simulink model "Protection"  (R2023b)
settings: Solver=FixedStepAuto  StartTime=0.0  StopTime=2  RelTol=1e-3
InitFcn:
  | Ts_Control=100e-6;
  | fs=50000;
  | Ts=1/fs/10;
  | Ts_Power=Ts;
  | Ts_control=5*Ts;
  | wnom=314.16;
  | Lf=5e-3;
  | Rf=0.1;
  | Cf=50e-6;
  | 
  | 
  | % choosing crossover frequency
  | fc=(1/10)*fs;
  | wc=2*pi*fc;
  | Ti=1/wc;
  | Kpc=Lf/Ti;
  | 
  | Kic=Rf/Ti;
  | 
  | x=[837.555 8.2389 0.057896 268.1361 0.74685 242.918 0.062838 291.0935]
  | 
  | 
  | Kvi=x(1);Kvp=x(2);Kcp=x(3);Kci=x(4);
  | Kvpb=x(5);Kvib=x(6);Kcpb=x(7);Kcib=x(8);
  | 
  | 
  | x1=[0.202905850069502  0.158544693742674   0.10408       75.97091  837.555350377473 8.2389271001531  0.10408       75.97091];
  | 
  | Kvif=x1(1);Kvpf=x1(2);Kcpf=x1(3);Kcif=x1(4);
  | Kvim=x1(5);Kvpm=x1(6);Kcpm=x1(7);Kcim=x1(8);
undefined symbols (not defined in the file): D1, Delta, Hydride, Metal, Nickel, sigbuilder_block
libraries: spsSeriesRLCBranchLib x52, spsVoltageMeasurementLib x22, powerlib_extras x18, spsCurrentMeasurementLib x13, spsIdealSwitchLib x12, simulink x8, slpidlib x7, spsGroundLib x6, spsBreakerLib x5, spsDiodeLib x4, spsIGBTLib x4, spsThreePhaseVIMeasurementLib x4
(part 2 of 2)

== system Protection/PV 1/MPPT ==
  In1 : Inport
  In2 : Inport  Port=2
  Add1 : Sum  Inputs=-+
  Constant1 : Constant  Value=0
  Constant2 : Constant  Value=0.5
  Constant3 : Constant
  MPPT : Subsystem
  Relational Operator : RelationalOperator  Operator=<  OutDataTypeStr=boolean  InputSameDT=off
  Repeating Sequence : simulink/Sources/Repeating Sequence  rep_seq_t=[0 0.00005 0.0001]  rep_seq_y=[0 1 0]
  Sign : Signum
  Switch2 : Switch  Criteria=u2 > Threshold  SaturateOnIntegerOverflow=off  InputSameDT=off
  Unit Delay1 : UnitDelay  SampleTime=2e-6  HasFrameUpgradeWarning=on
  Unit Delay2 : UnitDelay  SampleTime=2e-6  HasFrameUpgradeWarning=on
  Out1 : Outport
  wires:
  Relational Operator/1 -> Out1/1
  Repeating Sequence/1 -> Relational Operator/2
  Add1/1 -> Relational Operator/1
  Constant2/1 -> Add1/2
  In2/1 -> Unit Delay2/1
  In1/1 -> Unit Delay1/1
  Switch2/1 -> Add1/1
  Constant3/1 -> Switch2/3
  Sign/1 -> Switch2/2
  Constant1/1 -> Switch2/1
  Unit Delay2/1 -> MPPT/2(I_PV)
  Unit Delay1/1 -> MPPT/1(V_PV)
  MPPT/1(sign) -> Sign/1

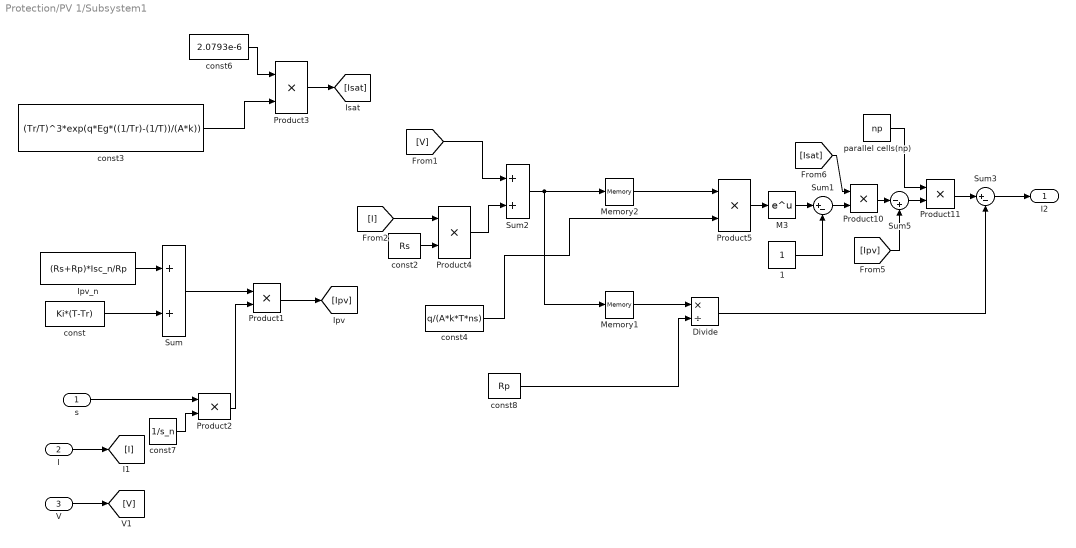
== system Protection/PV 1/Subsystem1 ==
  s : Inport
  I : Inport  Port=2
  V : Inport  Port=3
  1 : Constant
  Divide : Product  Inputs=*/
  Ipv_n : Constant  Value=(Rs+Rp)*Isc_n/Rp
  M3 : Math  SignedPower=on
  Memory1 : Memory
  Memory2 : Memory
  Product{1..5,10..11} (7 alike) : Product  RndMeth=Zero
  Sum : Sum
  Sum1 : Sum  Inputs=|+-
  Sum2 : Sum
  Sum3 : Sum  Inputs=|+-
  Sum5 : Sum  Inputs=|-+
  const : Constant  Value=Ki*(T-Tr)
  const2 : Constant  Value=Rs
  const3 : Constant  Value=(Tr/T)^3*exp(q*Eg*((1/Tr)-(1/T))/(A*k))
  const4 : Constant  Value=q/(A*k*T*ns)
  const6 : Constant  Value=2.0793e-6
  const7 : Constant  Value=1/s_n
  const8 : Constant  Value=Rp
  parallel cells(np) : Constant  Value=np
  I2 : Outport
  wires:
  Memory2/1 -> Product5/1
  Memory1/1 -> Divide/1
  Divide/1 -> Sum3/2
  Sum3/1 -> I2/1
  Product11/1 -> Sum3/1
  const8/1 -> Divide/2
  Ipv_n/1 -> Sum/1
  Product4/1 -> Sum2/2
  const7/1 -> Product2/2
  s/1 -> Product2/1
  Product2/1 -> Product1/2
  Sum2/1 -> Memory1/1, Memory2/1
  parallel cells(np)/1 -> Product11/1
  Sum5/1 -> Product11/2
  Product10/1 -> Sum5/1
  [Ipv] -> Sum5/2
  [Isat] -> Product10/1
  Sum1/1 -> Product10/2
  1/1 -> Sum1/2
  M3/1 -> Sum1/1
  Product5/1 -> M3/1
  const4/1 -> Product5/2
  [I] -> Product4/1
  const2/1 -> Product4/2
  [V] -> Sum2/1
  I/1 -> [I]
  V/1 -> [V]
  Product3/1 -> [Isat]
  const3/1 -> Product3/2
  Product1/1 -> [Ipv]
  Sum/1 -> Product1/1
  const/1 -> Sum/2
  const6/1 -> Product3/1

== system Protection/Subsystem/CPL1 ==
  2 : powerlib_extras/Control  Blocks/1st-Order  Filter  FilterType=Lowpass  Tc=2e-3  Initialize=off  Vac_Init=[0.8 -25 60]  Vdc_Init=-0.4  PlotResponse=off  param1=[1 500 1]
  Current Measurement : spsCurrentMeasurementLib/Current Measurement  PhasorSimulation=off  OutputType=Complex  PSBequivalent=0
  Diode1 : spsDiodeLib/Diode  Ron=0.001  Lon=0  Vf=0.8  IC=0  UseSnubber=off  Rs=500  Cs=250e-9  Measurements=off
  Display2 : Display
  Display3 : Display
  Display4 : Display
  IGBT : spsIGBTLib/IGBT  Ron=0.001  Lon=0  Vf=1  Tf=1e-6  Tt=2e-6  IC=0  Rs=1e5  Cs=inf  Measurements=on
  Product1 : Product  RndMeth=Zero
  SLB : spsSeriesRLCBranchLib/Series RLC Branch  LConnTagsString=__new0  RConnTagsString=__new0  BranchType=RL  Resistance=0.01  Inductance=9.2e-3  SetiL0=off  InitialCurrent=0  Capacitance=1e-6  Setx0=off  InitialVoltage=0  Measurements=Branch current
  Scope2 : Scope  NumInputPorts=2
  Subsystem : Subsystem
  Terminator : Terminator
  Unit Delay : UnitDelay  SampleTime=-1  HasFrameUpgradeWarning=on
  Voltage Measurement : spsVoltageMeasurementLib/Voltage Measurement  PhasorSimulation=off  OutputType=Complex  PSBequivalent=0
  Voltage Measurement1 : spsVoltageMeasurementLib/Voltage Measurement  PhasorSimulation=off  OutputType=Complex  PSBequivalent=0
  dc link1 : spsSeriesRLCBranchLib/Series RLC Branch  LConnTagsString=__new0  RConnTagsString=__new0  BranchType=C  Resistance=1  Inductance=1e-3  SetiL0=off  InitialCurrent=0  Capacitance=5000e-6  Setx0=on  InitialVoltage=240  Measurements=None
  Vout+ : PMIOPort  Tag=PMCPort  Side=Right
  Vout_ : PMIOPort  Tag=PMCPort  Port=2  Side=Right
  +Vin : PMIOPort  Tag=PMCPort  Port=3  Side=Left
  _Vin : PMIOPort  Tag=PMCPort  Port=4  Side=Left
  wires:
  Voltage Measurement1/1 -> Display4/1
  IGBT/1 -> Terminator/1
  Current Measurement/1 -> Subsystem/1(IL), Display3/1, Product1/2
  Voltage Measurement/1 -> Product1/1, Scope2/1, Subsystem/2(Vdc), Display2/1
  Subsystem/1(Out2) -> Unit Delay/1
  Unit Delay/1 -> IGBT/1
  Product1/1 -> 2/1
  2/1 -> Scope2/2
  connections:
  Diode1/LConn1 -- _Vin/RConn1 -- Voltage Measurement1/LConn2 -- Voltage Measurement/LConn2 -- Vout_/RConn1 -- dc link1/RConn1
  Current Measurement/LConn1 -- SLB/RConn1
  IGBT/RConn1 -- Diode1/RConn1 -- SLB/LConn1
  dc link1/LConn1 -- Current Measurement/RConn1 -- Voltage Measurement/LConn1 -- Vout+/RConn1
  Voltage Measurement1/LConn1 -- IGBT/LConn1 -- +Vin/RConn1

== system Protection/Subsystem1/CPL1 ==
  2 : powerlib_extras/Control  Blocks/1st-Order  Filter  FilterType=Lowpass  Tc=2e-3  Initialize=off  Vac_Init=[0.8 -25 60]  Vdc_Init=-0.4  PlotResponse=off  param1=[1 500 1]
  Current Measurement : spsCurrentMeasurementLib/Current Measurement  PhasorSimulation=off  OutputType=Complex  PSBequivalent=0
  Diode1 : spsDiodeLib/Diode  Ron=0.001  Lon=0  Vf=0.8  IC=0  UseSnubber=off  Rs=500  Cs=250e-9  Measurements=off
  Display2 : Display
  Display3 : Display
  Display4 : Display
  IGBT : spsIGBTLib/IGBT  Ron=0.001  Lon=0  Vf=1  Tf=1e-6  Tt=2e-6  IC=0  Rs=1e5  Cs=inf  Measurements=on
  Product1 : Product  RndMeth=Zero
  SLB : spsSeriesRLCBranchLib/Series RLC Branch  LConnTagsString=__new0  RConnTagsString=__new0  BranchType=RL  Resistance=0.01  Inductance=9.2e-3  SetiL0=off  InitialCurrent=0  Capacitance=1e-6  Setx0=off  InitialVoltage=0  Measurements=Branch current
  Scope2 : Scope  NumInputPorts=2
  Subsystem : Subsystem
  Terminator : Terminator
  Unit Delay : UnitDelay  SampleTime=-1  HasFrameUpgradeWarning=on
  Voltage Measurement : spsVoltageMeasurementLib/Voltage Measurement  PhasorSimulation=off  OutputType=Complex  PSBequivalent=0
  Voltage Measurement1 : spsVoltageMeasurementLib/Voltage Measurement  PhasorSimulation=off  OutputType=Complex  PSBequivalent=0
  dc link1 : spsSeriesRLCBranchLib/Series RLC Branch  LConnTagsString=__new0  RConnTagsString=__new0  BranchType=C  Resistance=1  Inductance=1e-3  SetiL0=off  InitialCurrent=0  Capacitance=5000e-6  Setx0=on  InitialVoltage=240  Measurements=None
  Vout+ : PMIOPort  Tag=PMCPort  Side=Right
  Vout_ : PMIOPort  Tag=PMCPort  Port=2  Side=Right
  +Vin : PMIOPort  Tag=PMCPort  Port=3  Side=Left
  _Vin : PMIOPort  Tag=PMCPort  Port=4  Side=Left
  wires:
  Voltage Measurement1/1 -> Display4/1
  IGBT/1 -> Terminator/1
  Current Measurement/1 -> Subsystem/1(IL), Display3/1, Product1/2
  Voltage Measurement/1 -> Product1/1, Scope2/1, Subsystem/2(Vdc), Display2/1
  Subsystem/1(Out2) -> Unit Delay/1
  Unit Delay/1 -> IGBT/1
  Product1/1 -> 2/1
  2/1 -> Scope2/2
  connections:
  Diode1/LConn1 -- _Vin/RConn1 -- Voltage Measurement1/LConn2 -- Voltage Measurement/LConn2 -- Vout_/RConn1 -- dc link1/RConn1
  Current Measurement/LConn1 -- SLB/RConn1
  IGBT/RConn1 -- Diode1/RConn1 -- SLB/LConn1
  dc link1/LConn1 -- Current Measurement/RConn1 -- Voltage Measurement/LConn1 -- Vout+/RConn1
  Voltage Measurement1/LConn1 -- IGBT/LConn1 -- +Vin/RConn1

== system Protection/Subsystem4/LC Filter1 ==
  "0.15 mH " : spsThreePhaseSeriesRLCBranchLib/Three-Phase Series RLC Branch  LConnTagsString=A|B|C  RConnTagsString=A|B|C  BranchType=RL  Resistance=Rf  Inductance=Lf  Capacitance=1.0  Measurements=None
  C1 : spsSeriesRLCBranchLib/Series RLC Branch  LConnTagsString=__new0  RConnTagsString=__new0  BranchType=C  Resistance=1.0  Inductance=1.0  SetiL0=off  InitialCurrent=0  Capacitance=Cf  Setx0=on  InitialVoltage=415  Measurements=Branch voltage
  C2 : spsSeriesRLCBranchLib/Series RLC Branch  LConnTagsString=__new0  RConnTagsString=__new0  BranchType=C  Resistance=1.0  Inductance=1.0  SetiL0=off  InitialCurrent=0  Capacitance=Cf  Setx0=on  InitialVoltage=415  Measurements=Branch voltage
  C3 : spsSeriesRLCBranchLib/Series RLC Branch  LConnTagsString=__new0  RConnTagsString=__new0  BranchType=C  Resistance=1.0  Inductance=1.0  SetiL0=off  InitialCurrent=0  Capacitance=Cf  Setx0=on  InitialVoltage=415  Measurements=Branch voltage
  Ground : spsGroundLib/Ground  LConnTagsString=a
  A : PMIOPort  Side=Left
  B : PMIOPort  Port=2  Side=Left
  C : PMIOPort  Port=3  Side=Left
  "A " : PMIOPort  Port=4  Side=Right
  "B " : PMIOPort  Port=5  Side=Right
  "C " : PMIOPort  Port=6  Side=Right
  connections:
  B/RConn1 -- "0.15 mH "/LConn2
  A/RConn1 -- "0.15 mH "/LConn1
  C/RConn1 -- "0.15 mH "/LConn3
  "A "/RConn1 -- C1/LConn1 -- "0.15 mH "/RConn1
  "B "/RConn1 -- "0.15 mH "/RConn2 -- C2/LConn1
  "C "/RConn1 -- C3/LConn1 -- "0.15 mH "/RConn3
  C1/RConn1 -- C3/RConn1 -- Ground/LConn1 -- C2/RConn1

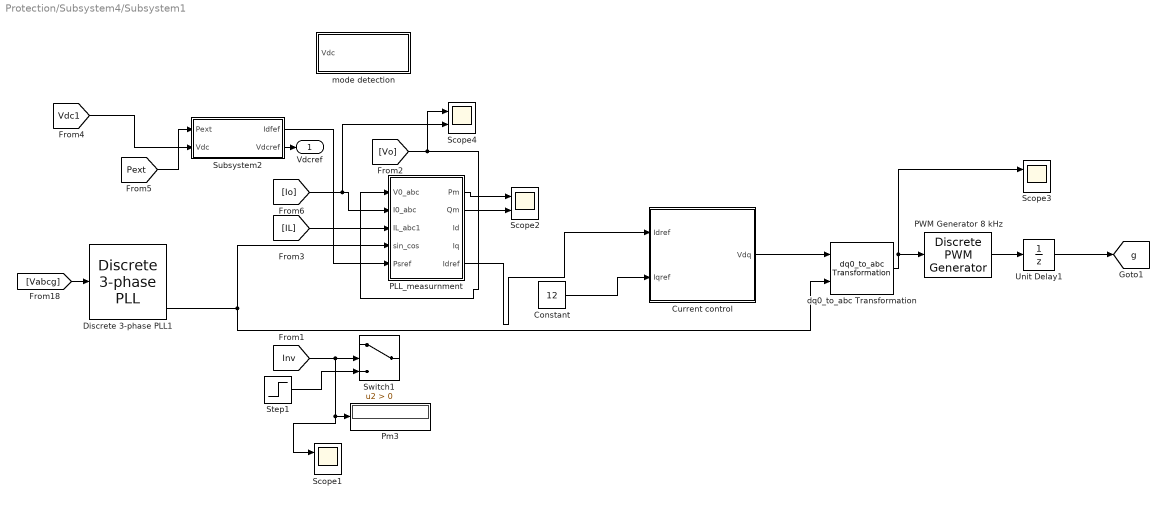
== system Protection/Subsystem4/Subsystem1 ==
  Constant : Constant  Value=12
  Current control : Subsystem
  Discrete 3-phase PLL1 : powerlib_extras/Discrete  Control Blocks/Discrete 3-phase PLL  Fmin=40  Par_Init=[0 50]  ParK=[ 180 3200 1 ]  Ts=Ts  AGC=on
  PLL_measurnment : Subsystem
  PWM Generator 8 kHz : powerlib_extras/Discrete  Control Blocks/Discrete PWM Generator  GeneratorMode="3-arm  bridge (6 pulses)"  Fc=fs  Ts=Ts  Internal=off  mIndex=0.4  Freq=50  Phase=0
  Pm3 : Display
  Scope{1..4} (4 alike) : Scope  NumInputPorts=2
  Step1 : Step  Time=0.2  After=0  SampleTime=0
  Subsystem2 : Subsystem
  Switch1 : Switch  Criteria=u2 > Threshold  SaturateOnIntegerOverflow=off  InputSameDT=off
  Unit Delay1 : UnitDelay  SampleTime=Ts  HasFrameUpgradeWarning=on
  dq0_to_abc Transformation : powerlib_extras/Measurements/dq0_to_abc Transformation
  mode detection : Subsystem
  Vdcref : Outport
  tag scope: g=global
  wires:
  [Io] -> Scope4/2, PLL_measurnment/2(I0_abc)
  PLL_measurnment/2(Qm) -> Scope2/2
  [Vabcg] -> Discrete 3-phase PLL1/1
  PLL_measurnment/1(Pm) -> Scope2/1
  Constant/1 -> Current control/2(Iqref)
  [Vo] -> Scope4/1, PLL_measurnment/1(V0_abc)
  [IL] -> PLL_measurnment/3(IL_abc1)
  [Pext] -> Subsystem2/1(Pext)
  Subsystem2/2(Vdcref) -> Vdcref/1
  Step1/1 -> Switch1/3
  [Inv] -> Scope1/1, Pm3/1, Switch1/2
  PLL_measurnment/5(Idref) -> Current control/1(Idref)
  Current control/1(Vdq) -> dq0_to_abc Transformation/1
  Unit Delay1/1 -> [g]
  dq0_to_abc Transformation/1 -> Scope3/1, PWM Generator 8 kHz/1
  PWM Generator 8 kHz/1 -> Unit Delay1/1
  Discrete 3-phase PLL1/3 -> PLL_measurnment/4(sin_cos), dq0_to_abc Transformation/2
  Subsystem2/1(Idfef) -> PLL_measurnment/5(Psref)
  [Vdc1] -> Subsystem2/2(Vdc)

== system Protection/PV /MPPT/MPPT ==
  V_PV : Inport
  I_PV : Inport  Port=2
  Add1 : Sum  Inputs=|++
  Add2 : Sum  Inputs=+-
  Add3 : Sum  Inputs=+-
  Compare To Zero : simulink/Logic and Bit Operations/Compare To Zero  relop=~=  OutDataTypeStr=uint8
  Constant2 : Constant  Value=1e-6
  Saturation : Saturate  UpperLimit=inf  LowerLimit=eps
  Switch2 : Switch  Criteria=u2 ~= 0  SaturateOnIntegerOverflow=off  InputSameDT=off
  Unit Delay : UnitDelay  SampleTime=-1  HasFrameUpgradeWarning=on
  Unit Delay1 : UnitDelay  SampleTime=-1  HasFrameUpgradeWarning=on
  div1 : Product  Inputs=*/  RndMeth=Zero
  div2 : Product  Inputs=*/  RndMeth=Zero
  sign : Outport
  wires:
  Add1/1 -> sign/1  "error"
  div2/1 -> Add1/2  "I/V"
  Saturation/1 -> div2/2
  Add2/1 -> div1/1  "dI"
  Add3/1 -> Switch2/1, Compare To Zero/1  "dV"
  Unit Delay/1 -> Add2/2
  I_PV/1 -> Add2/1, Unit Delay/1, div2/1  "I"
  Constant2/1 -> Switch2/3
  Switch2/1 -> div1/2
  Compare To Zero/1 -> Switch2/2
  Unit Delay1/1 -> Add3/2
  div1/1 -> Add1/1  "dI/dV"
  V_PV/1 -> Saturation/1, Unit Delay1/1, Add3/1  "V"

== system Protection/PV 1/MPPT/MPPT ==
  V_PV : Inport
  I_PV : Inport  Port=2
  Add1 : Sum  Inputs=|++
  Add2 : Sum  Inputs=+-
  Add3 : Sum  Inputs=+-
  Compare To Zero : simulink/Logic and Bit Operations/Compare To Zero  relop=~=  OutDataTypeStr=uint8
  Constant2 : Constant  Value=1e-6
  Saturation : Saturate  UpperLimit=inf  LowerLimit=eps
  Switch2 : Switch  Criteria=u2 ~= 0  SaturateOnIntegerOverflow=off  InputSameDT=off
  Unit Delay : UnitDelay  SampleTime=-1  HasFrameUpgradeWarning=on
  Unit Delay1 : UnitDelay  SampleTime=-1  HasFrameUpgradeWarning=on
  div1 : Product  Inputs=*/  RndMeth=Zero
  div2 : Product  Inputs=*/  RndMeth=Zero
  sign : Outport
  wires:
  V_PV/1 -> Add3/1, Unit Delay1/1, Saturation/1  "V"
  div1/1 -> Add1/1  "dI/dV"
  Unit Delay1/1 -> Add3/2
  Compare To Zero/1 -> Switch2/2
  Switch2/1 -> div1/2
  Constant2/1 -> Switch2/3
  I_PV/1 -> div2/1, Unit Delay/1, Add2/1  "I"
  Unit Delay/1 -> Add2/2
  Add3/1 -> Compare To Zero/1, Switch2/1  "dV"
  Add2/1 -> div1/1  "dI"
  Saturation/1 -> div2/2
  div2/1 -> Add1/2  "I/V"
  Add1/1 -> sign/1  "error"

== system Protection/Subsystem/CPL1/Subsystem ==
  IL : Inport
  Vdc : Inport  Port=2
  Add1 : Sum  Inputs=+-
  Add4 : Sum  Inputs=-+
  Display1 : Display
  Display2 : Display
  Display5 : Display
  Memory1 : Memory
  Memory2 : Memory
  PID Controller : slpidlib/PID Controller  Controller=PI  Form=Parallel  TimeDomain=Discrete-time  UseExternalTs=off  SampleTime=10*2e-6  IntegratorMethod=Backward Euler  FilterMethod=Forward Euler  ControllerParametersSource=internal  P=0.062838  I=291.0935  UseKiTs=off  D=0  N=100  UseFilter=on  TunerSelectOption=Transfer Function Based (PID Tuner App)  InitialConditionSource=internal  InitialConditionForIntegrator=0  InitialConditionForFilter=0  DifferentiatorICPrevScaledInput=0  ExternalReset=none  TrackingMode=off  Kt=1  LimitOutput=on  SatLimitsSource=internal  UpperSaturationLimit=1  LowerSaturationLimit=0  LinearizeAsGain=on  AntiWindupMode=none  Kb=1  LimitIntegrator=off  UpperIntegratorSaturationLimit=inf  LowerIntegratorSaturationLimit=-inf  POutMin=[]  POutMax=[]  IOutMin=[]  IOutMax=[]  DOutMin=[]  DOutMax=[]  NOutMin=[]  NOutMax=[]  SumOutMin=[]  SumOutMax=[]  SaturationOutMin=[]  SaturationOutMax=[]  PParamMin=[]  PParamMax=[]  IParamMin=[]  IParamMax=[]  DParamMin=[]  DParamMax=[]  NParamMin=[]  NParamMax=[]  KbParamMin=[]  KbParamMax=[]  KtParamMin=[]  KtParamMax=[]  KbOutMin=[]  KbOutMax=[]  KtOutMin=[]  KtOutMax=[]  IntegratorOutMin=[]  IntegratorOutMax=[]  FilterOutMin=[]  FilterOutMax=[]  SumI1OutMin=[]  SumI1OutMax=[]  SumI2OutMin=[]  SumI2OutMax=[]  SumI3OutMin=[]  SumI3OutMax=[]  SumI4OutMin=[]  SumI4OutMax=[]  SumDOutMin=[]  SumDOutMax=[]  DifferentiatorOutMin=[]  DifferentiatorOutMax=[]  FilterDiffOutCoefMin=[]  FilterDiffOutCoefMax=[]  ReciprocalOutMin=[]  ReciprocalOutMax=[]  SumDenOutMin=[]  SumDenOutMax=[]  SumNumOutMin=[]  SumNumOutMax=[]  DivideOutMin=[]  DivideOutMax=[]  UdiffTsProdOutMin=[]  UdiffTsProdOutMax=[]  NTsProdOutMin=[]  NTsProdOutMax=[]  UintegralTsProdOutMin=[]  UintegralTsProdOutMax=[]  UngainTsProdOutMin=[]  UngainTsProdOutMax=[]  ClampingZeroOutDataTypeStr=Inherit: Inherit via back propagation  ClampingZeroOutMin=[]  ClampingZeroOutMax=[]  FilterDenConstantOutDataTypeStr=Inherit: Inherit via back propagation  FilterDenConstantOutMin=[]  FilterDenConstantOutMax=[]  PCopyOutDataTypeStr=Inherit: Inherit via back propagation  PCopyOutMin=[]  PCopyOutMax=[]  NCopyOutDataTypeStr=Inherit: Inherit via back propagation  NCopyOutMin=[]  NCopyOutMax=[]  IntegratorContinuousStateAttributes=''  IntegratorStateMustResolveToSignalObject=off  IntegratorRTWStateStorageClass=Auto  FilterContinuousStateAttributes=''  FilterStateMustResolveToSignalObject=off  FilterRTWStateStorageClass=Auto  ParallelPVariant=InternalParameters  IdealPVariant=Disabled  IVariant=InternalParameters  DVariant=Disabled  IntegratorVariant=Discrete  SatVariant=Enabled  AWVariant=Passthrough  PCopyVariant=Disabled  TRVariant=Disabled  FdbkBlocksVariant=Forward  IdealPFdbkVariant=Disabled  SatFdbkVariant=Disabled  DerivativeFilterVariant=Disabled  NVariant=Disabled  NCopyVariant=Disabled_SignalSpec  FilterICVariant=Disabled  IntegratorICVariant=InternalICs  ExternalResetVariant=Disabled  TRSumVariant=Passthrough  SumFdbkVariant=Disabled  SumVariant=Sum_PI  TsampFilterVariant=InternalTs  TsampNgainVariant=Passthrough  TsampIntegralVariant=Disabled_SignalSpec  ExternalSaturationOutDataTypeStr=Inherit: Same as second input
  PID Controller1 : slpidlib/PID Controller  Controller=PI  Form=Parallel  TimeDomain=Discrete-time  UseExternalTs=off  SampleTime=10*2e-6  IntegratorMethod=Backward Euler  FilterMethod=Forward Euler  ControllerParametersSource=internal  P=0.74685  I=242.918  UseKiTs=off  D=0  N=100  UseFilter=on  TunerSelectOption=Transfer Function Based (PID Tuner App)  InitialConditionSource=internal  InitialConditionForIntegrator=0  InitialConditionForFilter=0  DifferentiatorICPrevScaledInput=0  ExternalReset=none  TrackingMode=off  Kt=1  LimitOutput=on  SatLimitsSource=internal  UpperSaturationLimit=50  LowerSaturationLimit=0  LinearizeAsGain=on  AntiWindupMode=none  Kb=1  LimitIntegrator=off  UpperIntegratorSaturationLimit=inf  LowerIntegratorSaturationLimit=-inf  POutMin=[]  POutMax=[]  IOutMin=[]  IOutMax=[]  DOutMin=[]  DOutMax=[]  NOutMin=[]  NOutMax=[]  SumOutMin=[]  SumOutMax=[]  SaturationOutMin=[]  SaturationOutMax=[]  PParamMin=[]  PParamMax=[]  IParamMin=[]  IParamMax=[]  DParamMin=[]  DParamMax=[]  NParamMin=[]  NParamMax=[]  KbParamMin=[]  KbParamMax=[]  KtParamMin=[]  KtParamMax=[]  KbOutMin=[]  KbOutMax=[]  KtOutMin=[]  KtOutMax=[]  IntegratorOutMin=[]  IntegratorOutMax=[]  FilterOutMin=[]  FilterOutMax=[]  SumI1OutMin=[]  SumI1OutMax=[]  SumI2OutMin=[]  SumI2OutMax=[]  SumI3OutMin=[]  SumI3OutMax=[]  SumI4OutMin=[]  SumI4OutMax=[]  SumDOutMin=[]  SumDOutMax=[]  DifferentiatorOutMin=[]  DifferentiatorOutMax=[]  FilterDiffOutCoefMin=[]  FilterDiffOutCoefMax=[]  ReciprocalOutMin=[]  ReciprocalOutMax=[]  SumDenOutMin=[]  SumDenOutMax=[]  SumNumOutMin=[]  SumNumOutMax=[]  DivideOutMin=[]  DivideOutMax=[]  UdiffTsProdOutMin=[]  UdiffTsProdOutMax=[]  NTsProdOutMin=[]  NTsProdOutMax=[]  UintegralTsProdOutMin=[]  UintegralTsProdOutMax=[]  UngainTsProdOutMin=[]  UngainTsProdOutMax=[]  ClampingZeroOutDataTypeStr=Inherit: Inherit via back propagation  ClampingZeroOutMin=[]  ClampingZeroOutMax=[]  FilterDenConstantOutDataTypeStr=Inherit: Inherit via back propagation  FilterDenConstantOutMin=[]  FilterDenConstantOutMax=[]  PCopyOutDataTypeStr=Inherit: Inherit via back propagation  PCopyOutMin=[]  PCopyOutMax=[]  NCopyOutDataTypeStr=Inherit: Inherit via back propagation  NCopyOutMin=[]  NCopyOutMax=[]  IntegratorContinuousStateAttributes=''  IntegratorStateMustResolveToSignalObject=off  IntegratorRTWStateStorageClass=Auto  FilterContinuousStateAttributes=''  FilterStateMustResolveToSignalObject=off  FilterRTWStateStorageClass=Auto  ParallelPVariant=InternalParameters  IdealPVariant=Disabled  IVariant=InternalParameters  DVariant=Disabled  IntegratorVariant=Discrete  SatVariant=Enabled  AWVariant=Passthrough  PCopyVariant=Disabled  TRVariant=Disabled  FdbkBlocksVariant=Forward  IdealPFdbkVariant=Disabled  SatFdbkVariant=Disabled  DerivativeFilterVariant=Disabled  NVariant=Disabled  NCopyVariant=Disabled_SignalSpec  FilterICVariant=Disabled  IntegratorICVariant=InternalICs  ExternalResetVariant=Disabled  TRSumVariant=Passthrough  SumFdbkVariant=Disabled  SumVariant=Sum_PI  TsampFilterVariant=InternalTs  TsampNgainVariant=Passthrough  TsampIntegralVariant=Disabled_SignalSpec  ExternalSaturationOutDataTypeStr=Inherit: Same as second input
  PWM Generator (DC-DC) : spsPWMGeneratorDCDCLib/PWM Generator (DC-DC)  Fsw=10000  Ts=2e-6
  Scope4 : Scope
  power3 : Constant  Value=240
  Out2 : Outport
  wires:
  Add4/1 -> PID Controller1/1, Display2/1
  Add1/1 -> Display5/1, PID Controller/1
  Memory2/1 -> Add1/2
  power3/1 -> Add4/2
  PID Controller/1 -> PWM Generator (DC-DC)/1, Scope4/1
  PID Controller1/1 -> Memory1/1
  Memory1/1 -> Add1/1
  Vdc/1 -> Add4/1
  IL/1 -> Display1/1, Memory2/1
  PWM Generator (DC-DC)/1 -> Out2/1

== system Protection/Subsystem1/CPL1/Subsystem ==
  IL : Inport
  Vdc : Inport  Port=2
  Add1 : Sum  Inputs=+-
  Add4 : Sum  Inputs=-+
  Display1 : Display
  Display2 : Display
  Display5 : Display
  Memory1 : Memory
  Memory2 : Memory
  Memory3 : Memory  InitialCondition=240
  PID Controller : slpidlib/PID Controller  Controller=PI  Form=Parallel  TimeDomain=Discrete-time  UseExternalTs=off  SampleTime=1*Ts  IntegratorMethod=Backward Euler  FilterMethod=Forward Euler  ControllerParametersSource=internal  P=Kcpb/2  I=Kcib  UseKiTs=off  D=0  N=100  UseFilter=on  TunerSelectOption=Transfer Function Based (PID Tuner App)  InitialConditionSource=internal  InitialConditionForIntegrator=0  InitialConditionForFilter=0  DifferentiatorICPrevScaledInput=0  ExternalReset=none  TrackingMode=off  Kt=1  LimitOutput=on  SatLimitsSource=internal  UpperSaturationLimit=1  LowerSaturationLimit=0  LinearizeAsGain=on  AntiWindupMode=none  Kb=1  LimitIntegrator=off  UpperIntegratorSaturationLimit=inf  LowerIntegratorSaturationLimit=-inf  POutMin=[]  POutMax=[]  IOutMin=[]  IOutMax=[]  DOutMin=[]  DOutMax=[]  NOutMin=[]  NOutMax=[]  SumOutMin=[]  SumOutMax=[]  SaturationOutMin=[]  SaturationOutMax=[]  PParamMin=[]  PParamMax=[]  IParamMin=[]  IParamMax=[]  DParamMin=[]  DParamMax=[]  NParamMin=[]  NParamMax=[]  KbParamMin=[]  KbParamMax=[]  KtParamMin=[]  KtParamMax=[]  KbOutMin=[]  KbOutMax=[]  KtOutMin=[]  KtOutMax=[]  IntegratorOutMin=[]  IntegratorOutMax=[]  FilterOutMin=[]  FilterOutMax=[]  SumI1OutMin=[]  SumI1OutMax=[]  SumI2OutMin=[]  SumI2OutMax=[]  SumI3OutMin=[]  SumI3OutMax=[]  SumI4OutMin=[]  SumI4OutMax=[]  SumDOutMin=[]  SumDOutMax=[]  DifferentiatorOutMin=[]  DifferentiatorOutMax=[]  FilterDiffOutCoefMin=[]  FilterDiffOutCoefMax=[]  ReciprocalOutMin=[]  ReciprocalOutMax=[]  SumDenOutMin=[]  SumDenOutMax=[]  SumNumOutMin=[]  SumNumOutMax=[]  DivideOutMin=[]  DivideOutMax=[]  UdiffTsProdOutMin=[]  UdiffTsProdOutMax=[]  NTsProdOutMin=[]  NTsProdOutMax=[]  UintegralTsProdOutMin=[]  UintegralTsProdOutMax=[]  UngainTsProdOutMin=[]  UngainTsProdOutMax=[]  ClampingZeroOutDataTypeStr=Inherit: Inherit via back propagation  ClampingZeroOutMin=[]  ClampingZeroOutMax=[]  FilterDenConstantOutDataTypeStr=Inherit: Inherit via back propagation  FilterDenConstantOutMin=[]  FilterDenConstantOutMax=[]  PCopyOutDataTypeStr=Inherit: Inherit via back propagation  PCopyOutMin=[]  PCopyOutMax=[]  NCopyOutDataTypeStr=Inherit: Inherit via back propagation  NCopyOutMin=[]  NCopyOutMax=[]  IntegratorContinuousStateAttributes=''  IntegratorStateMustResolveToSignalObject=off  IntegratorRTWStateStorageClass=Auto  FilterContinuousStateAttributes=''  FilterStateMustResolveToSignalObject=off  FilterRTWStateStorageClass=Auto  ParallelPVariant=InternalParameters  IdealPVariant=Disabled  IVariant=InternalParameters  DVariant=Disabled  IntegratorVariant=Discrete  SatVariant=Enabled  AWVariant=Passthrough  PCopyVariant=Disabled  TRVariant=Disabled  FdbkBlocksVariant=Forward  IdealPFdbkVariant=Disabled  SatFdbkVariant=Disabled  DerivativeFilterVariant=Disabled  NVariant=Disabled  NCopyVariant=Disabled_SignalSpec  FilterICVariant=Disabled  IntegratorICVariant=InternalICs  ExternalResetVariant=Disabled  TRSumVariant=Passthrough  SumFdbkVariant=Disabled  SumVariant=Sum_PI  TsampFilterVariant=InternalTs  TsampNgainVariant=Passthrough  TsampIntegralVariant=Disabled_SignalSpec  ExternalSaturationOutDataTypeStr=Inherit: Same as second input
  PID Controller1 : slpidlib/PID Controller  Controller=PI  Form=Parallel  TimeDomain=Discrete-time  UseExternalTs=off  SampleTime=1*Ts  IntegratorMethod=Backward Euler  FilterMethod=Forward Euler  ControllerParametersSource=internal  P=Kvpb  I=Kvib  UseKiTs=off  D=0  N=100  UseFilter=on  TunerSelectOption=Transfer Function Based (PID Tuner App)  InitialConditionSource=internal  InitialConditionForIntegrator=0  InitialConditionForFilter=0  DifferentiatorICPrevScaledInput=0  ExternalReset=none  TrackingMode=off  Kt=1  LimitOutput=on  SatLimitsSource=internal  UpperSaturationLimit=50  LowerSaturationLimit=0  LinearizeAsGain=on  AntiWindupMode=none  Kb=1  LimitIntegrator=off  UpperIntegratorSaturationLimit=inf  LowerIntegratorSaturationLimit=-inf  POutMin=[]  POutMax=[]  IOutMin=[]  IOutMax=[]  DOutMin=[]  DOutMax=[]  NOutMin=[]  NOutMax=[]  SumOutMin=[]  SumOutMax=[]  SaturationOutMin=[]  SaturationOutMax=[]  PParamMin=[]  PParamMax=[]  IParamMin=[]  IParamMax=[]  DParamMin=[]  DParamMax=[]  NParamMin=[]  NParamMax=[]  KbParamMin=[]  KbParamMax=[]  KtParamMin=[]  KtParamMax=[]  KbOutMin=[]  KbOutMax=[]  KtOutMin=[]  KtOutMax=[]  IntegratorOutMin=[]  IntegratorOutMax=[]  FilterOutMin=[]  FilterOutMax=[]  SumI1OutMin=[]  SumI1OutMax=[]  SumI2OutMin=[]  SumI2OutMax=[]  SumI3OutMin=[]  SumI3OutMax=[]  SumI4OutMin=[]  SumI4OutMax=[]  SumDOutMin=[]  SumDOutMax=[]  DifferentiatorOutMin=[]  DifferentiatorOutMax=[]  FilterDiffOutCoefMin=[]  FilterDiffOutCoefMax=[]  ReciprocalOutMin=[]  ReciprocalOutMax=[]  SumDenOutMin=[]  SumDenOutMax=[]  SumNumOutMin=[]  SumNumOutMax=[]  DivideOutMin=[]  DivideOutMax=[]  UdiffTsProdOutMin=[]  UdiffTsProdOutMax=[]  NTsProdOutMin=[]  NTsProdOutMax=[]  UintegralTsProdOutMin=[]  UintegralTsProdOutMax=[]  UngainTsProdOutMin=[]  UngainTsProdOutMax=[]  ClampingZeroOutDataTypeStr=Inherit: Inherit via back propagation  ClampingZeroOutMin=[]  ClampingZeroOutMax=[]  FilterDenConstantOutDataTypeStr=Inherit: Inherit via back propagation  FilterDenConstantOutMin=[]  FilterDenConstantOutMax=[]  PCopyOutDataTypeStr=Inherit: Inherit via back propagation  PCopyOutMin=[]  PCopyOutMax=[]  NCopyOutDataTypeStr=Inherit: Inherit via back propagation  NCopyOutMin=[]  NCopyOutMax=[]  IntegratorContinuousStateAttributes=''  IntegratorStateMustResolveToSignalObject=off  IntegratorRTWStateStorageClass=Auto  FilterContinuousStateAttributes=''  FilterStateMustResolveToSignalObject=off  FilterRTWStateStorageClass=Auto  ParallelPVariant=InternalParameters  IdealPVariant=Disabled  IVariant=InternalParameters  DVariant=Disabled  IntegratorVariant=Discrete  SatVariant=Enabled  AWVariant=Passthrough  PCopyVariant=Disabled  TRVariant=Disabled  FdbkBlocksVariant=Forward  IdealPFdbkVariant=Disabled  SatFdbkVariant=Disabled  DerivativeFilterVariant=Disabled  NVariant=Disabled  NCopyVariant=Disabled_SignalSpec  FilterICVariant=Disabled  IntegratorICVariant=InternalICs  ExternalResetVariant=Disabled  TRSumVariant=Passthrough  SumFdbkVariant=Disabled  SumVariant=Sum_PI  TsampFilterVariant=InternalTs  TsampNgainVariant=Passthrough  TsampIntegralVariant=Disabled_SignalSpec  ExternalSaturationOutDataTypeStr=Inherit: Same as second input
  PWM Generator (DC-DC) : spsPWMGeneratorDCDCLib/PWM Generator (DC-DC)  Fsw=10000  Ts=Ts
  Scope4 : Scope
  power3 : Constant  Value=240
  Out2 : Outport
  wires:
  Add4/1 -> PID Controller1/1, Display2/1
  Add1/1 -> Display5/1, PID Controller/1
  Memory2/1 -> Add1/2
  power3/1 -> Add4/2
  PID Controller/1 -> PWM Generator (DC-DC)/1, Scope4/1
  PID Controller1/1 -> Memory1/1
  Memory1/1 -> Add1/1
  Vdc/1 -> Memory3/1
  IL/1 -> Display1/1, Memory2/1
  PWM Generator (DC-DC)/1 -> Out2/1
  Memory3/1 -> Add4/1

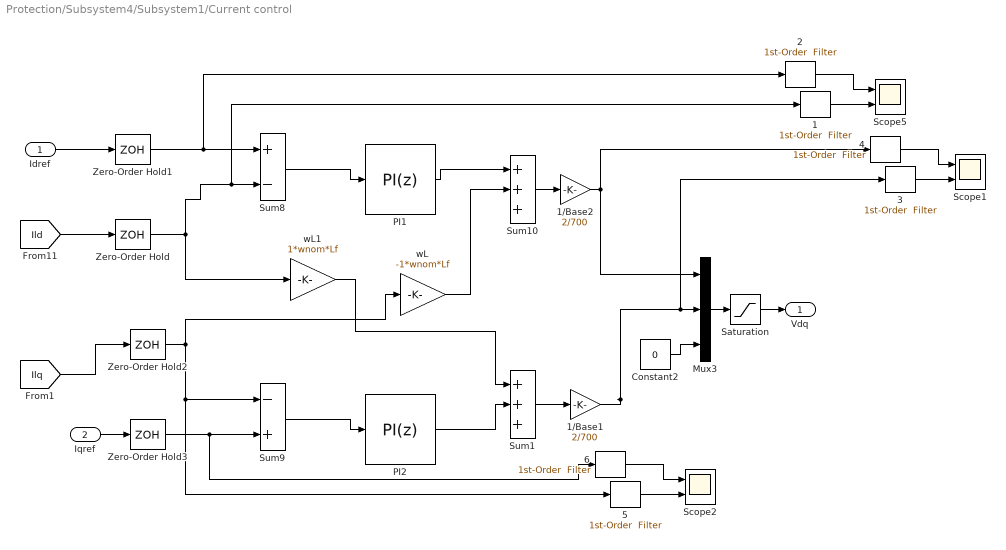
== system Protection/Subsystem4/Subsystem1/Current control ==
  Idref : Inport
  Iqref : Inport  Port=2
  {1..6} (6 alike) : powerlib_extras/Control  Blocks/1st-Order  Filter  FilterType=Lowpass  Tc=2e-3  Initialize=off  Vac_Init=[0.8 -25 60]  Vdc_Init=-0.4  PlotResponse=off  param1=[1 500 1]
  1/Base1 : Gain  Gain=2/700
  1/Base2 : Gain  Gain=2/700
  Constant2 : Constant  Value=0
  Mux3 : Mux  Inputs=3
  PI1 : slpidlib/PID Controller  Controller=PI  Form=Parallel  TimeDomain=Discrete-time  UseExternalTs=off  SampleTime=Ts_control  IntegratorMethod=Forward Euler  FilterMethod=Forward Euler  ControllerParametersSource=internal  P=Kpc  I=Kic  UseKiTs=off  D=0  N=100  UseFilter=on  TunerSelectOption=Transfer Function Based (PID Tuner App)  InitialConditionSource=internal  InitialConditionForIntegrator=0  InitialConditionForFilter=0  DifferentiatorICPrevScaledInput=0  ExternalReset=none  TrackingMode=off  Kt=1  LimitOutput=on  SatLimitsSource=internal  UpperSaturationLimit=400  LowerSaturationLimit=-400  LinearizeAsGain=off  AntiWindupMode=clamping  Kb=1  LimitIntegrator=off  UpperIntegratorSaturationLimit=inf  LowerIntegratorSaturationLimit=-inf  POutMin=[]  POutMax=[]  IOutMin=[]  IOutMax=[]  DOutMin=[]  DOutMax=[]  NOutMin=[]  NOutMax=[]  SumOutMin=[]  SumOutMax=[]  SaturationOutMin=[]  SaturationOutMax=[]  PParamMin=[]  PParamMax=[]  IParamMin=[]  IParamMax=[]  DParamMin=[]  DParamMax=[]  NParamMin=[]  NParamMax=[]  KbParamMin=[]  KbParamMax=[]  KtParamMin=[]  KtParamMax=[]  KbOutMin=[]  KbOutMax=[]  KtOutMin=[]  KtOutMax=[]  IntegratorOutMin=[]  IntegratorOutMax=[]  FilterOutMin=[]  FilterOutMax=[]  SumI1OutMin=[]  SumI1OutMax=[]  SumI2OutMin=[]  SumI2OutMax=[]  SumI3OutMin=[]  SumI3OutMax=[]  SumI4OutMin=[]  SumI4OutMax=[]  SumDOutMin=[]  SumDOutMax=[]  DifferentiatorOutMin=[]  DifferentiatorOutMax=[]  FilterDiffOutCoefMin=[]  FilterDiffOutCoefMax=[]  ReciprocalOutMin=[]  ReciprocalOutMax=[]  SumDenOutMin=[]  SumDenOutMax=[]  SumNumOutMin=[]  SumNumOutMax=[]  DivideOutMin=[]  DivideOutMax=[]  UdiffTsProdOutMin=[]  UdiffTsProdOutMax=[]  NTsProdOutMin=[]  NTsProdOutMax=[]  UintegralTsProdOutMin=[]  UintegralTsProdOutMax=[]  UngainTsProdOutMin=[]  UngainTsProdOutMax=[]  ClampingZeroOutDataTypeStr=Inherit: Inherit via back propagation  ClampingZeroOutMin=[]  ClampingZeroOutMax=[]  FilterDenConstantOutDataTypeStr=Inherit: Inherit via back propagation  FilterDenConstantOutMin=[]  FilterDenConstantOutMax=[]  PCopyOutDataTypeStr=Inherit: Inherit via back propagation  PCopyOutMin=[]  PCopyOutMax=[]  NCopyOutDataTypeStr=Inherit: Inherit via back propagation  NCopyOutMin=[]  NCopyOutMax=[]  IntegratorContinuousStateAttributes=''  IntegratorStateMustResolveToSignalObject=off  IntegratorRTWStateStorageClass=Auto  FilterContinuousStateAttributes=''  FilterStateMustResolveToSignalObject=off  FilterRTWStateStorageClass=Auto  ParallelPVariant=InternalParameters  IdealPVariant=Disabled  IVariant=InternalParameters  DVariant=Disabled  IntegratorVariant=Discrete  SatVariant=Enabled  AWVariant=DiscClampingParallel  PCopyVariant=Disabled  TRVariant=Disabled  FdbkBlocksVariant=Forward  IdealPFdbkVariant=Disabled  SatFdbkVariant=Disabled  DerivativeFilterVariant=Disabled  NVariant=Disabled  NCopyVariant=Disabled_SignalSpec  FilterICVariant=Disabled  IntegratorICVariant=InternalICs  ExternalResetVariant=Disabled  TRSumVariant=Passthrough  SumFdbkVariant=Disabled  SumVariant=Sum_PI  TsampFilterVariant=InternalTs  TsampNgainVariant=Passthrough  TsampIntegralVariant=Disabled_SignalSpec  ExternalSaturationOutDataTypeStr=Inherit: Same as second input
  PI2 : slpidlib/PID Controller  Controller=PI  Form=Parallel  TimeDomain=Discrete-time  UseExternalTs=off  SampleTime=Ts_control  IntegratorMethod=Forward Euler  FilterMethod=Forward Euler  ControllerParametersSource=internal  P=Kpc  I=Kic  UseKiTs=off  D=0  N=100  UseFilter=on  TunerSelectOption=Transfer Function Based (PID Tuner App)  InitialConditionSource=internal  InitialConditionForIntegrator=0  InitialConditionForFilter=0  DifferentiatorICPrevScaledInput=0  ExternalReset=none  TrackingMode=off  Kt=1  LimitOutput=on  SatLimitsSource=internal  UpperSaturationLimit=600  LowerSaturationLimit=-600  LinearizeAsGain=off  AntiWindupMode=clamping  Kb=1  LimitIntegrator=off  UpperIntegratorSaturationLimit=inf  LowerIntegratorSaturationLimit=-inf  POutMin=[]  POutMax=[]  IOutMin=[]  IOutMax=[]  DOutMin=[]  DOutMax=[]  NOutMin=[]  NOutMax=[]  SumOutMin=[]  SumOutMax=[]  SaturationOutMin=[]  SaturationOutMax=[]  PParamMin=[]  PParamMax=[]  IParamMin=[]  IParamMax=[]  DParamMin=[]  DParamMax=[]  NParamMin=[]  NParamMax=[]  KbParamMin=[]  KbParamMax=[]  KtParamMin=[]  KtParamMax=[]  KbOutMin=[]  KbOutMax=[]  KtOutMin=[]  KtOutMax=[]  IntegratorOutMin=[]  IntegratorOutMax=[]  FilterOutMin=[]  FilterOutMax=[]  SumI1OutMin=[]  SumI1OutMax=[]  SumI2OutMin=[]  SumI2OutMax=[]  SumI3OutMin=[]  SumI3OutMax=[]  SumI4OutMin=[]  SumI4OutMax=[]  SumDOutMin=[]  SumDOutMax=[]  DifferentiatorOutMin=[]  DifferentiatorOutMax=[]  FilterDiffOutCoefMin=[]  FilterDiffOutCoefMax=[]  ReciprocalOutMin=[]  ReciprocalOutMax=[]  SumDenOutMin=[]  SumDenOutMax=[]  SumNumOutMin=[]  SumNumOutMax=[]  DivideOutMin=[]  DivideOutMax=[]  UdiffTsProdOutMin=[]  UdiffTsProdOutMax=[]  NTsProdOutMin=[]  NTsProdOutMax=[]  UintegralTsProdOutMin=[]  UintegralTsProdOutMax=[]  UngainTsProdOutMin=[]  UngainTsProdOutMax=[]  ClampingZeroOutDataTypeStr=Inherit: Inherit via back propagation  ClampingZeroOutMin=[]  ClampingZeroOutMax=[]  FilterDenConstantOutDataTypeStr=Inherit: Inherit via back propagation  FilterDenConstantOutMin=[]  FilterDenConstantOutMax=[]  PCopyOutDataTypeStr=Inherit: Inherit via back propagation  PCopyOutMin=[]  PCopyOutMax=[]  NCopyOutDataTypeStr=Inherit: Inherit via back propagation  NCopyOutMin=[]  NCopyOutMax=[]  IntegratorContinuousStateAttributes=''  IntegratorStateMustResolveToSignalObject=off  IntegratorRTWStateStorageClass=Auto  FilterContinuousStateAttributes=''  FilterStateMustResolveToSignalObject=off  FilterRTWStateStorageClass=Auto  ParallelPVariant=InternalParameters  IdealPVariant=Disabled  IVariant=InternalParameters  DVariant=Disabled  IntegratorVariant=Discrete  SatVariant=Enabled  AWVariant=DiscClampingParallel  PCopyVariant=Disabled  TRVariant=Disabled  FdbkBlocksVariant=Forward  IdealPFdbkVariant=Disabled  SatFdbkVariant=Disabled  DerivativeFilterVariant=Disabled  NVariant=Disabled  NCopyVariant=Disabled_SignalSpec  FilterICVariant=Disabled  IntegratorICVariant=InternalICs  ExternalResetVariant=Disabled  TRSumVariant=Passthrough  SumFdbkVariant=Disabled  SumVariant=Sum_PI  TsampFilterVariant=InternalTs  TsampNgainVariant=Passthrough  TsampIntegralVariant=Disabled_SignalSpec  ExternalSaturationOutDataTypeStr=Inherit: Same as second input
  Saturation : Saturate  UpperLimit=1  LowerLimit=-1
  Scope1 : Scope  NumInputPorts=2
  Scope2 : Scope  NumInputPorts=2
  Scope5 : Scope  NumInputPorts=2
  Sum1 : Sum  Inputs=+++
  Sum10 : Sum  Inputs=+++
  Sum8 : Sum  Inputs=+-
  Sum9 : Sum  Inputs=-+
  Zero-Order Hold{,1..3} (4 alike) : ZeroOrderHold  SampleTime=Ts
  wL : Gain  Gain=-1*wnom*Lf
  wL1 : Gain  Gain=1*wnom*Lf
  Vdq : Outport
  wires:
  Sum8/1 -> PI1/1
  Sum9/1 -> PI2/1
  PI2/1 -> Sum1/2
  PI1/1 -> Sum10/1
  wL/1 -> Sum10/2
  wL1/1 -> Sum1/1
  Sum10/1 -> 1/Base2/1
  Mux3/1 -> Saturation/1
  Sum1/1 -> 1/Base1/1
  Idref/1 -> Zero-Order Hold1/1
  [Ild] -> Zero-Order Hold/1
  2/1 -> Scope5/1
  1/1 -> Scope5/2
  1/Base2/1 -> Mux3/1, 4/1
  1/Base1/1 -> 3/1, Mux3/2
  Saturation/1 -> Vdq/1
  4/1 -> Scope1/1
  3/1 -> Scope1/2
  Iqref/1 -> Zero-Order Hold3/1
  [Ilq] -> Zero-Order Hold2/1
  6/1 -> Scope2/1
  5/1 -> Scope2/2
  Constant2/1 -> Mux3/3
  Zero-Order Hold/1 -> 1/1, Sum8/2, wL1/1
  Zero-Order Hold1/1 -> 2/1, Sum8/1
  Zero-Order Hold2/1 -> 5/1, Sum9/1, wL/1
  ? -> ?
  Zero-Order Hold3/1 -> 6/1, Sum9/2

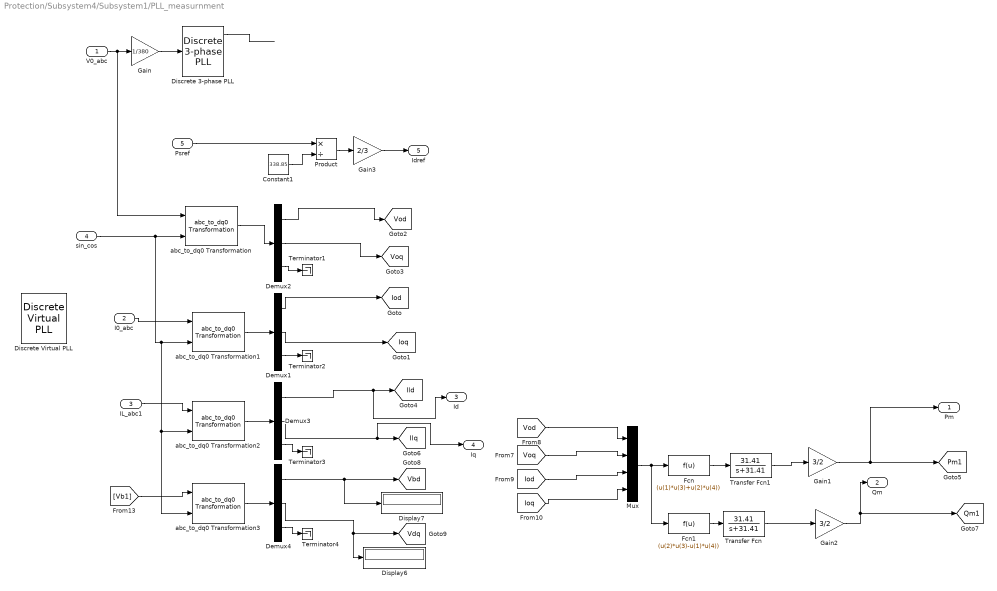
== system Protection/Subsystem4/Subsystem1/PLL_measurnment ==
  V0_abc : Inport
  I0_abc : Inport  Port=2
  IL_abc1 : Inport  Port=3
  sin_cos : Inport  Port=4
  Psref : Inport  Port=5
  Constant1 : Constant  Value=338.85
  Demux{1..4} (4 alike) : Demux  Outputs=3
  Discrete 3-phase PLL : powerlib_extras/Discrete  Control Blocks/Discrete 3-phase PLL  Fmin=50  Par_Init=[0 50]  ParK=[ 180 3200 1 ]  Ts=Ts  AGC=off
  Discrete Virtual PLL : powerlib_extras/Discrete  Control Blocks/Discrete Virtual PLL  Freq=50  Phase=0  Ts=Ts
  Display6 : Display
  Display7 : Display
  Fcn : Fcn  Expr=(u(1)*u(3)+u(2)*u(4))
  Fcn1 : Fcn  Expr=(u(2)*u(3)-u(1)*u(4))
  Gain : Gain  Gain=1/380
  Gain1 : Gain  Gain=3/2
  Gain2 : Gain  Gain=3/2
  Gain3 : Gain  Gain=2/3
  Mux : Mux
  Product : Product  Inputs=*/
  Terminator{1..4} (4 alike) : Terminator
  Transfer Fcn : TransferFcn  Numerator=[0 31.41]  Denominator=[1 31.41]
  Transfer Fcn1 : TransferFcn  Numerator=[0 31.41]  Denominator=[1 31.41]
  abc_to_dq0 Transformation{,1..3} (4 alike) : powerlib_extras/Measurements/abc_to_dq0 Transformation
  Pm : Outport
  Qm : Outport  Port=2
  Id : Outport  Port=3
  Iq : Outport  Port=4
  Idref : Outport  Port=5
  tag scope: Ild=global, Ilq=global, Iod=global, Ioq=global, Pm1=global, Qm1=global, Vbd=global, Vdq=global, Vod=global, Voq=global
  wires:
  Discrete 3-phase PLL/1 -> ?
  V0_abc/1 -> Gain/1, abc_to_dq0 Transformation/1
  abc_to_dq0 Transformation/1 -> Demux2/1
  Gain/1 -> Discrete 3-phase PLL/1
  I0_abc/1 -> abc_to_dq0 Transformation1/1
  abc_to_dq0 Transformation1/1 -> Demux1/1
  IL_abc1/1 -> abc_to_dq0 Transformation2/1
  Demux2/3 -> Terminator1/1
  Demux1/3 -> Terminator2/1
  Demux3/3 -> Terminator3/1
  [Vod] -> Mux/1
  [Voq] -> Mux/2
  [Iod] -> Mux/3
  [Ioq] -> Mux/4
  Mux/1 -> Fcn/1, Fcn1/1
  Fcn1/1 -> Transfer Fcn/1
  Fcn/1 -> Transfer Fcn1/1
  Transfer Fcn1/1 -> Gain1/1
  Transfer Fcn/1 -> Gain2/1
  Demux1/1 -> [Iod]
  Demux1/2 -> [Ioq]
  Demux3/2 -> Iq/1, [Ilq]
  Demux2/1 -> [Vod]
  Demux2/2 -> [Voq]
  Demux3/1 -> Id/1, [Ild]
  abc_to_dq0 Transformation2/1 -> Demux3/1
  sin_cos/1 -> abc_to_dq0 Transformation/2, abc_to_dq0 Transformation1/2, abc_to_dq0 Transformation3/2, abc_to_dq0 Transformation2/2
  [Vb1] -> abc_to_dq0 Transformation3/1
  Demux4/3 -> Terminator4/1
  Demux4/2 -> Display6/1, [Vdq]
  Demux4/1 -> Display7/1, [Vbd]
  abc_to_dq0 Transformation3/1 -> Demux4/1
  Gain1/1 -> [Pm1], Pm/1
  Gain2/1 -> [Qm1], Qm/1
  Product/1 -> Gain3/1
  Psref/1 -> Product/1
  Gain3/1 -> Idref/1
  Constant1/1 -> Product/2

== system Protection/Subsystem4/Subsystem1/Subsystem2 ==
  Pext : Inport
  Vdc : Inport  Port=2
  Constant1 : Constant  Value=10000
  Constant2 : Constant  Value=700
  Gain : Gain  Gain=-1
  Gain1 : Gain  Gain=0.005
  Kv : TransferFcn  Numerator=[6.996e05 1.596e07]  Denominator=[1 1.772e05 0]
  Product : Product
  Product1 : Product  Inputs=*/
  Saturation : Saturate  UpperLimit=1e6  LowerLimit=-1e6
  Subsystem1 : Subsystem
  Subsystem2 : Subsystem
  Sum : Sum  Inputs=|-+
  Sum1 : Sum  Inputs=|+-
  Sum2 : Sum  Inputs=|++
  Zero-Order Hold1 : ZeroOrderHold  SampleTime=Ts
  Idfef : Outport
  Vdcref : Outport  Port=2
  wires:
  Product/1 -> Sum/1
  Pext/1 -> Subsystem1/2(Pext)
  Sum/1 -> Gain/1
  Subsystem1/1(Psref) -> Idfef/1
  Kv/1 -> Sum2/1
  Constant1/1 -> Product1/1
  Gain1/1 -> Sum1/2
  Constant2/1 -> Subsystem1/3(Vref), Vdcref/1
  [Iext] -> Gain1/1
  Vdc/1 -> Saturation/1, Zero-Order Hold1/1
  Zero-Order Hold1/1 -> Subsystem1/1(Vdc)
  Saturation/1 -> Product1/2

== system Protection/Subsystem4/Subsystem1/mode detection ==
  Vdc : Inport
  Compare To Constant : simulink/Logic and Bit Operations/Compare To Constant  relop=>  const=0.05  OutDataTypeStr=boolean
  Compare To Constant1 : simulink/Logic and Bit Operations/Compare To Constant  relop=<  const=-0.05  OutDataTypeStr=boolean
  Compare To Zero : simulink/Logic and Bit Operations/Compare To Zero  relop=>  OutDataTypeStr=boolean
  Compare To Zero1 : simulink/Logic and Bit Operations/Compare To Zero  relop=<  OutDataTypeStr=boolean
  Constant : Constant  Value=700
  Constant1 : Constant  Value=0
  Gain : Gain  Gain=1/700
  Logical Operator : Logic  Operator=OR  AllPortsSameDT=off  OutDataTypeStr=boolean
  Logical Operator1 : Logic  Operator=NOT  AllPortsSameDT=off  OutDataTypeStr=boolean
  Pm1 : Display
  Pm2 : Display
  Sum : Sum  Inputs=|-+
  Switch : Switch  Criteria=u2 > Threshold  SaturateOnIntegerOverflow=off  InputSameDT=off
  Switch1 : Switch  Criteria=u2 > Threshold  SaturateOnIntegerOverflow=off  InputSameDT=off
  tag scope: Bat=global, Inv=global
  wires:
  Constant/1 -> Sum/2
  Vdc/1 -> Sum/1
  Sum/1 -> Gain/1
  Compare To Zero/1 -> Switch/2
  Switch/1 -> Compare To Constant/1
  Gain/1 -> Pm1/1, Switch1/1, Compare To Zero1/1, Switch/1, Compare To Zero/1
  Compare To Zero1/1 -> Switch1/2
  Switch1/1 -> Compare To Constant1/1
  Constant1/1 -> Switch1/3, Switch/3
  Compare To Constant/1 -> Logical Operator/1
  Compare To Constant1/1 -> Logical Operator/2
  Logical Operator/1 -> Pm2/1, Logical Operator1/1, [Bat]
  Logical Operator1/1 -> [Inv]

== system Protection/Subsystem4/Subsystem1/Subsystem2/Subsystem1 ==
  Vdc : Inport
  Pext : Inport  Port=2
  Vref : Inport  Port=3
  Discrete Transfer Fcn : DiscreteTransferFcn  Numerator=[0.0242 1.28e-05 -0.02419]  Denominator="[1 -1.928  0.928]"  SampleTime=Ts
  Gain : Gain  Gain=-1
  Product : Product
  Product1 : Product
  Saturation : Saturate  UpperLimit=100e3  LowerLimit=-100e3
  Sum : Sum  Inputs=|-+
  Sum2 : Sum  Inputs=|++
  Psref : Outport
  wires:
  Product/1 -> Sum/1
  Product1/1 -> Sum/2
  Sum/1 -> Gain/1
  Pext/1 -> Sum2/2
  Sum2/1 -> Saturation/1
  Saturation/1 -> Psref/1
  Gain/1 -> Discrete Transfer Fcn/1
  Discrete Transfer Fcn/1 -> Sum2/1
  Vref/1 -> Product1/1, Product1/2
  Vdc/1 -> Product/2, Product/1

== system Protection/Subsystem4/Subsystem1/Subsystem2/Subsystem2 ==
  Vdcref : Inport
  Pext : Inport  Port=2
  Vdc : Inport  Port=3
  Subsystem2 : Subsystem
  Psref : Outport
  wires:
  Pext/1 -> Subsystem2/2(Pext)
  Subsystem2/1(Psref) -> Psref/1
  Vdcref/1 -> Subsystem2/3(Vdcref1)
  Vdc/1 -> Subsystem2/1(Vdc)

== system Protection/Subsystem4/Subsystem1/Subsystem2/Subsystem2/Subsystem2 ==
  Vdc : Inport
  Pext : Inport  Port=2
  Vdcref1 : Inport  Port=3
  Discrete Transfer Fcn : DiscreteTransferFcn  Numerator="[1.684  0.0002401  -1.684]"  Denominator=[1 -1.757 0.7568]
  Gain : Gain  Gain=-1
  Product : Product
  Product1 : Product
  Saturation : Saturate  UpperLimit=100e3  LowerLimit=-100e3
  Sum : Sum  Inputs=|-+
  Sum2 : Sum  Inputs=|++
  Zero-Order Hold1 : ZeroOrderHold  SampleTime=Ts
  Psref : Outport
  wires:
  Product/1 -> Sum/1
  Vdc/1 -> Zero-Order Hold1/1
  Product1/1 -> Sum/2
  Sum/1 -> Gain/1
  Pext/1 -> Sum2/2
  Sum2/1 -> Saturation/1
  Saturation/1 -> Psref/1
  Gain/1 -> Discrete Transfer Fcn/1
  Discrete Transfer Fcn/1 -> Sum2/1
  Vdcref1/1 -> Product1/1, Product1/2
  Zero-Order Hold1/1 -> Product/2, Product/1
